simulink model "NNN_pick_and_place_without_camera"  (R2022b)
settings: Solver=ode4  StartTime=0.0  StopTime=inf  FixedStep=1/500  RelTol=1e-3  EnableMultiTasking=on
InitFcn:
  | % Positions
  | home = [0; 0.49; 0.45];
  | pick = [0.49; 0; 0.45];
  | place = [-0.3; -0.3; 0.05];
  | 
  | % Liste des cibles : On alterne juste entre Pick et Place
  | % Le format doit être : [x1 y1 z1; x2 y2 z2; ...]
  | waypoints = [pick'; place'];
  | 
  | % Vitesse désirée (m/s) - Remplace la durée fixe
  | robot_speed = 0.4;
  | 
  | % Temps de pause (secondes)
  | wait_time_home = 2; % Temps de repos avant le pick and place
  | wait_time_pick = 2 ;  % Temps pour attraper
  | wait_time_place = 1 ; % Temps pour déposer
  | 
  | wait_times = [wait_time_home, wait_time_pick, wait_time_place];
undefined symbols (not defined in the file): HIL, qc_get_step_size, waypoints
libraries: quarc_library x8
settings Model: SimulationMode=external  ExtModeTrigDuration=10000  Creator=fvranes  LastModifiedBy=QARM2
settings SolverCC: AlgebraicLoopSolver=TrustRegion  PositivePriorityOrder=on
settings DataIOCC: SaveOutput=off  SignalLogging=off  DSMLogging=off  SaveTime=off  ReturnWorkspaceOutputs=off
settings DebuggingCC: UnconnectedInputMsg=warning  UnconnectedOutputMsg=warning  UnconnectedLineMsg=warning  SFMachineParentedDataDiag=warning  ArithmeticOperatorsInVariantConditions=warning
settings ModelReferenceCC: EnableRefExpFcnMdlSchedulingChecks=on
settings SFSimCC: SimUseLocalCustomCode=off  CustomCodeUndefinedFunction=UseInterfaceOnly
settings RTWCC: Description=QUARC Win64 Target Using Toolchain  SystemTargetFile=quarc_win64.tlc  TemplateMakefile=quarc_default_tmf  RTWUseLocalCustomCode=off  Toolchain=QUARC win64 | nmake (64-bit Windows)  BuildConfiguration=Faster Runs
settings CodeAppCC: StateflowObjectComments=on
settings STFCustomTargetCC: TargetLangStandard=C99 (ISO)  ConcurrentExecutionCompliant=on  GRTInterface=on  UseToolchainInfoCompliant=on  SystemTargetFile=quarc_win64.tlc
settings GRTTargetCC: ParMdlRefBuildCompliant=off  CompOptLevelCompliant=off  CombineOutputUpdateFcns=off  MatFileLogging=off  CPPClassGenCompliant=off  GRTInterface=on  ExtMode=on  ExtModeMexFile=quarc_comm
settings ConfigComp: CovMetricSettings=dswe

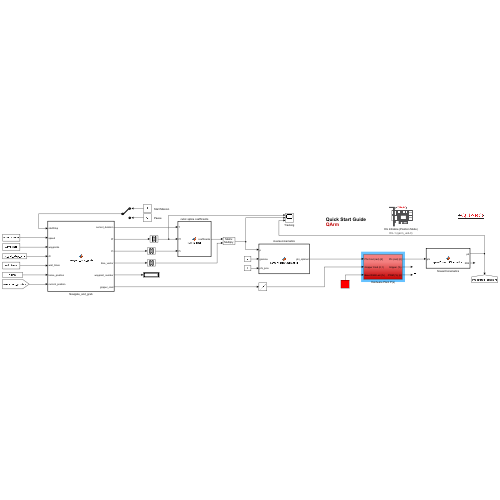
[thumbnail: Simulink's stored preview of the top-level diagram]
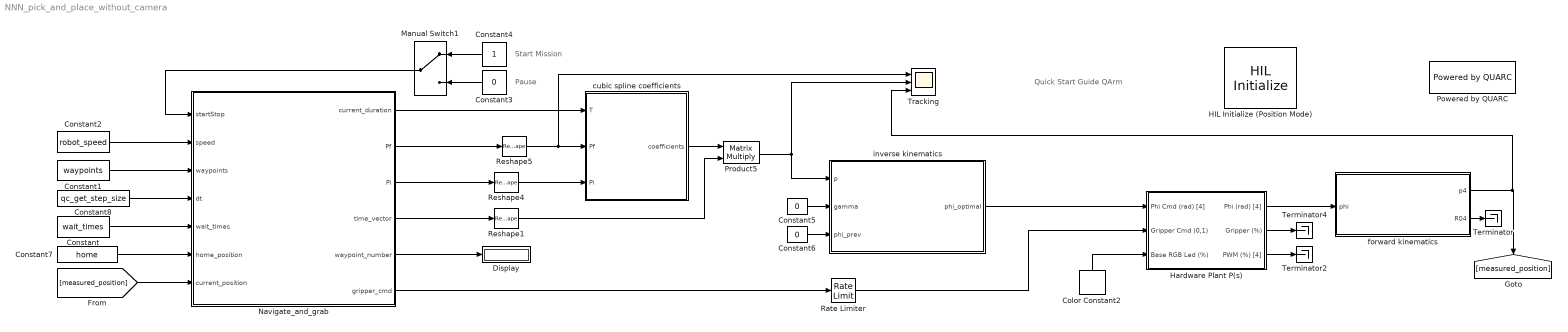
== system NNN_pick_and_place_without_camera ==
  note: Quick Start Guide
      | QArm
  note: Pause
  note: Start Mission
  Color Constant2 : quarc_library/Sources/Signals/Color Constant  color=[1 0 0]
      settings: SourceProductName=QUARC Targets
  Constant : Constant  Value=wait_times
  Constant1 : Constant  Value=waypoints  VectorParams1D=off
  Constant2 : Constant  Value=robot_speed
  Constant3 : Constant  Value=0
  Constant4 : Constant
  Constant5 : Constant  Value=0
  Constant6 : Constant  Value=0
  Constant7 : Constant  Value=home
  Constant8 : Constant  Value=qc_get_step_size
  Display : Display
  HIL Initialize (Position Mode) : quarc_library/Data Acquisition/Generic/Configuration/HIL Initialize  object_name=HIL-1  board_type=qarm_usb  board_number=0  board_options=j0_mode=0;j1_mode=0;j2_mode=0;j3_mode=0;gripper_mode=0;j0_profile_config=0;j0_profile_velocity=1.5708;j0_profile_acceleration=1.0472;j1_profile_config=0;j1_profile_velocity=1.5708;j1_profile_acceleration=1.0472;j2_profile_config=0;j2_profile_velocity=1.5708;j2_profile_acceleration=1.0472;j3_profile_config=0;j3_profile_velocity=1.5708;j3_profile_acceleration=1.0472;  exclusive=off  active=on  hardware_clocks=[0]  clock_modes=[]  initial_clock_frequencies=[]  set_clock_params_at_start=off  set_clock_params_at_switch_in=off  set_clock_frequencies_at_start=off  set_clock_frequencies_at_switch_in=off  analog_input_channels=[0:9]  analog_input_configurations=[]  analog_input_maximums=5  analog_input_minimums=0  set_analog_input_params_at_start=off  set_analog_input_params_at_switch_in=off  analog_output_channels=[]  analog_output_maximums=[]  analog_output_minimums=[]  initial_analog_outputs=[]  final_analog_outputs=[]  watchdog_analog_outputs=[]  set_analog_output_params_at_start=off  set_analog_output_params_at_switch_in=off  set_analog_outputs_at_start=off  set_analog_outputs_at_switch_in=off  set_analog_outputs_at_terminate=off  set_analog_outputs_at_switch_out=off  set_analog_outputs_on_watchdog=off  digital_input_channels=[]  digital_output_channels=[]  digital_output_configuration=[]  initial_digital_outputs=[0]  final_digital_outputs=[0]  watchdog_digital_outputs=[0]  set_digital_output_params_at_start=off  set_digital_output_params_at_switch_in=off  set_digital_outputs_at_start=on  set_digital_outputs_at_switch_in=off  set_digital_outputs_at_terminate=on  set_digital_outputs_at_switch_out=off  set_digital_outputs_on_watchdog=on  encoder_channels=[]  quadrature=[4]  encoder_filter_frequency=[]  initial_encoder_counts=[0]  set_encoder_params_at_start=off  set_encoder_params_at_switch_in=off  set_encoder_counts_at_start=on  set_encoder_counts_at_switch_in=off  pwm_channels=[]  pwm_modes=[0]  pwm_frequency=50  pwm_configuration=[0]  pwm_alignment=[0]  pwm_polarity=[1]  pwm_leading_deadband=[]  pwm_trailing_deadband=[]  initial_pwm_outputs=[0]  final_pwm_outputs=[0]  watchdog_pwm_outputs=[0]  set_pwm_params_at_start=on  set_pwm_params_at_switch_in=off  set_pwm_outputs_at_start=on  set_pwm_outputs_at_switch_in=off  set_pwm_outputs_at_terminate=on  set_pwm_outputs_at_switch_out=off  set_pwm_outputs_on_watchdog=on  other_output_channels=[1000:1004 11000:11008]  initial_other_outputs=[0]  final_other_outputs=[0]  watchdog_other_outputs=[0]  set_other_outputs_at_start=on  set_other_outputs_at_switch_in=off  set_other_outputs_at_terminate=on  set_other_outputs_at_switch_out=off  set_other_outputs_on_watchdog=on
  Hardware Plant P(s) : Subsystem
  Manual Switch1 : ManualSwitch
  Navigate_and_grab : MATLAB Function  TreatAsAtomicUnit=on
  Powered by QUARC : quarc_library/Logos/Powered by QUARC
  Product5 : Product  Multiplication=Matrix(*)
  Rate Limiter : RateLimiter  RisingSlewLimit=0.05
  Reshape1 : Reshape  OutputDimensionality=Column vector (2-D)
  Reshape4 : Reshape  OutputDimensionality=Column vector (2-D)
  Reshape5 : Reshape  OutputDimensionality=Column vector (2-D)
  Terminator : Terminator
  Terminator2 : Terminator
  Terminator4 : Terminator
  Tracking : Scope  NumInputPorts=3
  cubic spline coefficients : MATLAB Function  TreatAsAtomicUnit=on
  forward kinematics : MATLAB Function  TreatAsAtomicUnit=on
  inverse kinematics : MATLAB Function  TreatAsAtomicUnit=on
  wires:
  forward kinematics/2(R04) -> Terminator/1
  Hardware Plant P(s)/1(Phi (rad) [4]) -> forward kinematics/1(phi)
  Color Constant2/1 -> Hardware Plant P(s)/3(Base RGB Led (%))
  Rate Limiter/1 -> Hardware Plant P(s)/2(Gripper Cmd (0,1))
  Hardware Plant P(s)/3(PWM (%) [4]) -> Terminator2/1
  Hardware Plant P(s)/2(Gripper (%)) -> Terminator4/1
  inverse kinematics/1(phi_optimal) -> Hardware Plant P(s)/1(Phi Cmd (rad) [4])
  Constant1/1 -> Navigate_and_grab/3(waypoints)
  Navigate_and_grab/3(Pi) -> Reshape4/1
  Constant4/1 -> Manual Switch1/1
  Navigate_and_grab/4(time_vector) -> Reshape1/1
  cubic spline coefficients/1(coefficients) -> Product5/1
  Constant8/1 -> Navigate_and_grab/4(dt)
  Manual Switch1/1 -> Navigate_and_grab/1(startStop)
  Navigate_and_grab/2(Pf) -> Reshape5/1
  Constant3/1 -> Manual Switch1/2
  Constant2/1 -> Navigate_and_grab/2(speed)
  Reshape1/1 -> Product5/2
  Reshape4/1 -> cubic spline coefficients/3(Pi)
  Navigate_and_grab/5(waypoint_number) -> Display/1
  Reshape5/1 -> Tracking/1, cubic spline coefficients/2(Pf)
  Product5/1 -> Tracking/2, inverse kinematics/1(p)
  forward kinematics/1(p4) -> [measured_position], Tracking/3
  Constant5/1 -> inverse kinematics/2(gamma)
  Navigate_and_grab/1(current_duration) -> cubic spline coefficients/1(T)
  Navigate_and_grab/6(gripper_cmd) -> Rate Limiter/1
  Constant/1 -> Navigate_and_grab/5(wait_times)
  Constant7/1 -> Navigate_and_grab/6(home_position)
  [measured_position] -> Navigate_and_grab/7(current_position)
  Constant6/1 -> inverse kinematics/3(phi_prev)

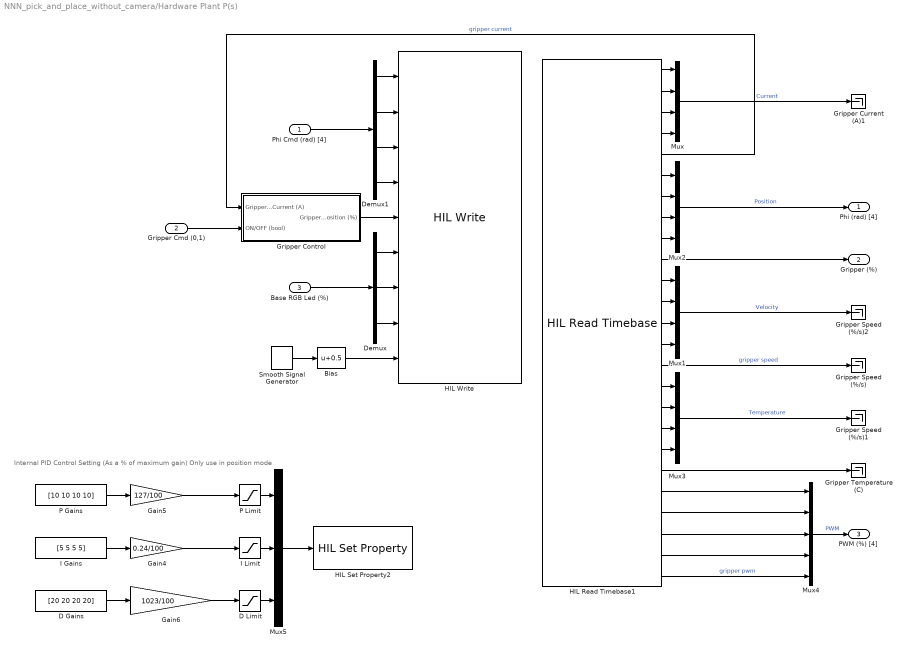
== system NNN_pick_and_place_without_camera/Hardware Plant P(s) ==
  note: Internal PID Control Setting (As a % of maximum gain)
      | Only use in position mode
  Phi Cmd (rad) [4] : Inport
  Gripper Cmd (0,1) : Inport  Port=2
  Base RGB Led (%) : Inport  Port=3
  Bias : Bias  Bias=0.5  SaturateOnIntegerOverflow=off
  D Gains : Constant  Value=[20 20 20 20]
  D Limit : Saturate  UpperLimit=[1023 1023 1023 1023]  LowerLimit=[0 0 0 0]
  Demux : Demux  Outputs=3
  Demux1 : Demux
  Gain4 : Gain  Gain=0.24/100
  Gain5 : Gain  Gain=127/100
  Gain6 : Gain  Gain=1023/100
  Gripper Control : Subsystem
  Gripper Current (A)1 : Terminator
  Gripper Speed (%/s) : Terminator
  Gripper Speed (%/s)1 : Terminator
  Gripper Speed (%/s)2 : Terminator
  Gripper Temperature (C) : Terminator
  HIL Read Timebase1 : quarc_library/Data Acquisition/Generic/Timebases/HIL Read Timebase  object_name=HIL-1  clock=0  analog_channels=[5:9]  encoder_channels=[]  digital_channels=[]  other_channels=[1000:1004 3000:3004 10000:10004 11000:11004]  active=on  vector_output=off  data_type_mode=Inherit via back propagation  encoder_data_type=double  digital_data_type=boolean  overflow_mode=Error on overflow  samples_in_buffer=max(ceil(1/qc_get_step_size), 1)
  HIL Set Property2 : quarc_library/Data Acquisition/Generic/Configuration/HIL Set Property  object_name=HIL-1  property_type=2  property_codes=[128:131 133:136 138:141]  property_source=2  property_value_num=0  set_at_start=on  sample_time=-1  active=off
      settings: AttributesFormatString=(%<object_name>)  SourceProductName=QUARC Targets
  HIL Write : quarc_library/Data Acquisition/Generic/Immediate I//O/HIL Write  object_name=HIL-1  analog_channels=[]  pwm_channels=[]  digital_channels=[]  other_channels=[1000:1004 11005:11008]  sample_time=-1  active=on  vector_input=off
  I Gains : Constant  Value=[5 5 5 5]
  I Limit : Saturate  UpperLimit=[0.24 0.24 0.24 0.24]  LowerLimit=[0 0 0 0]
  Mux{,1..3} (4 alike) : Mux
  Mux4 : Mux  Inputs=5
  Mux5 : Mux  Inputs=3
  P Gains : Constant  Value=[10 10 10 10]
  P Limit : Saturate  UpperLimit=[127 127 127 127]  LowerLimit=[0 0 0 0]
  Smooth Signal Generator : quarc_library/Sources/Signals/Smooth Signal Generator  signal_type=Sine  source=Internal (dialog parameters)  amplitude=0.5  frequency=60/72  initial_phase=0  sample_time=qc_get_step_size  output_cos=off
      settings: SourceProductName=QUARC Targets
  Phi (rad) [4] : Outport  VectorParamsAs1DForOutWhenUnconnected=off
  Gripper (%) : Outport  Port=2  VectorParamsAs1DForOutWhenUnconnected=off
  PWM (%) [4] : Outport  Port=3  VectorParamsAs1DForOutWhenUnconnected=off
  wires:
  HIL Read Timebase1/10 -> Gripper (%)/1
  Mux4/1 -> PWM (%) [4]/1  "PWM"
  HIL Read Timebase1/25 -> Mux4/5  "gripper pwm"
  HIL Read Timebase1/24 -> Mux4/4
  HIL Read Timebase1/23 -> Mux4/3
  HIL Read Timebase1/22 -> Mux4/2
  HIL Read Timebase1/21 -> Mux4/1
  Mux2/1 -> Phi (rad) [4]/1  "Position"
  Phi Cmd (rad) [4]/1 -> Demux1/1
  Demux1/4 -> HIL Write/4
  Demux1/3 -> HIL Write/3
  Demux1/2 -> HIL Write/2
  Demux1/1 -> HIL Write/1
  Base RGB Led (%)/1 -> Demux/1
  Mux3/1 -> Gripper Speed (%/s)1/1  "Temperature"
  Mux1/1 -> Gripper Speed (%/s)2/1  "Velocity"
  Mux/1 -> Gripper Current (A)1/1  "Current"
  HIL Read Timebase1/20 -> Gripper Temperature (C)/1
  HIL Read Timebase1/1 -> Mux/1
  HIL Read Timebase1/2 -> Mux/2
  HIL Read Timebase1/13 -> Mux1/3
  Demux/2 -> HIL Write/7
  HIL Read Timebase1/19 -> Mux3/4
  Demux/1 -> HIL Write/6
  HIL Read Timebase1/11 -> Mux1/1
  HIL Read Timebase1/16 -> Mux3/1
  HIL Read Timebase1/17 -> Mux3/2
  HIL Read Timebase1/3 -> Mux/3
  Demux/3 -> HIL Write/8
  HIL Read Timebase1/15 -> Gripper Speed (%/s)/1  "gripper speed"
  HIL Read Timebase1/5 -> Gripper Control/1(Gripper Current (A))  "gripper current"
  HIL Read Timebase1/7 -> Mux2/2
  HIL Read Timebase1/4 -> Mux/4
  HIL Read Timebase1/12 -> Mux1/2
  HIL Read Timebase1/8 -> Mux2/3
  HIL Read Timebase1/18 -> Mux3/3
  HIL Read Timebase1/6 -> Mux2/1
  HIL Read Timebase1/9 -> Mux2/4
  HIL Read Timebase1/14 -> Mux1/4
  Gripper Control/1(Gripper Position (%)) -> HIL Write/5
  Gripper Cmd (0,1)/1 -> Gripper Control/2(ON/OFF (bool))
  Smooth Signal Generator/1 -> Bias/1
  Bias/1 -> HIL Write/9
  P Limit/1 -> Mux5/1
  D Gains/1 -> Gain6/1
  D Limit/1 -> Mux5/3
  P Gains/1 -> Gain5/1
  Mux5/1 -> HIL Set Property2/1
  I Limit/1 -> Mux5/2
  Gain6/1 -> D Limit/1
  Gain5/1 -> P Limit/1
  Gain4/1 -> I Limit/1
  I Gains/1 -> Gain4/1

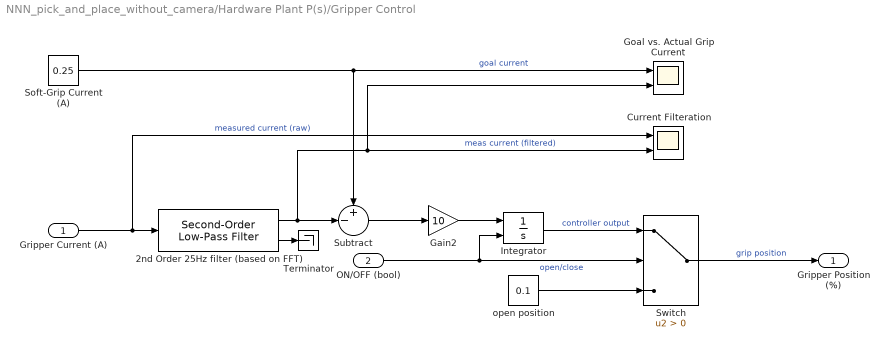
== system NNN_pick_and_place_without_camera/Hardware Plant P(s)/Gripper Control ==
  Gripper Current (A) : Inport
  ON/OFF (bool) : Inport  Port=2
  2nd Order 25Hz filter (based on FFT) : quarc_library/Continuous/Second-Order Low-Pass Filter  params_source=Internal (dialog parameters)  input_width=25*2*pi  input_zeta=1  input_init=0
  Current Filteration : Scope  NumInputPorts=2
  Gain2 : Gain  Gain=10
  Goal vs. Actual Grip Current : Scope  NumInputPorts=2
  Integrator : Integrator  ExternalReset=either  InitialCondition=0.1  LimitOutput=on  UpperSaturationLimit=0.9  LowerSaturationLimit=0.1
  Soft-Grip Current (A) : Constant  Value=0.25
  Subtract : Sum  Inputs=+-|
  Switch : Switch  Criteria=u2 > Threshold  SaturateOnIntegerOverflow=off  InputSameDT=off
  Terminator : Terminator
  open position : Constant  Value=0.1
  Gripper Position (%) : Outport  VectorParamsAs1DForOutWhenUnconnected=off
  wires:
  Gripper Current (A)/1 -> 2nd Order 25Hz filter (based on FFT)/1, Current Filteration/1  "measured current (raw)"
  ON/OFF (bool)/1 -> Switch/2, Integrator/2  "open/close"
  open position/1 -> Switch/3
  Switch/1 -> Gripper Position (%)/1  "grip position"
  Soft-Grip Current (A)/1 -> Subtract/1, Goal vs. Actual Grip Current/1  "goal current"
  2nd Order 25Hz filter (based on FFT)/1 -> Subtract/2, Current Filteration/2, Goal vs. Actual Grip Current/2  "meas current (filtered)"
  Subtract/1 -> Gain2/1
  Integrator/1 -> Switch/1  "controller output"
  Gain2/1 -> Integrator/1
  2nd Order 25Hz filter (based on FFT)/2 -> Terminator/1

== matlab function NNN_pick_and_place_without_camera/Navigate_and_grab ==
  data: startStop input; current_duration output; speed input; waypoints input; Pf output; dt input; wait_times input; home_position input; current_position input; Pi output; time_vector output; waypoint_number output; gripper_cmd output
function [current_duration, Pf, Pi, time_vector, waypoint_number, gripper_cmd] = navigate_and_grab(startStop, speed, waypoints, dt, wait_times, home_position, current_position)
    % MODIFICATION : Une seule entrée 'wait_times' à la fin au lieu de 3 séparées.
    % On suppose que wait_times = [Temps_Home, Temps_Pick, Temps_Place]

    %% Rising slew rate est la vitesse de fermeture
    %%falling slew rate est la vitesse d'ouverture

    %% 0. Lecture des temps (pour lisibilité)
    % C'est plus propre de les nommer ici que d'utiliser wait_times(1) partout
    TIME_HOME  = wait_times(1);
    TIME_PICK  = wait_times(2);
    TIME_PLACE = wait_times(3);

    %% 1. Initialisation
    persistent state          % 0:Vers Home, 1:Vers Waypoint, 2:Pause
    persistent p_start p_end  % Points
    persistent target_idx     % Index cible
    persistent t_clock        % Chrono
    persistent t_travel       % Durée voyage
    persistent t_wait         % Durée pause
    persistent grip_state     % État pince
    
    POSITION_TOLERANCE = 0.04; % 5 cm

    if isempty(state)
        state = 0;          
        p_start = current_position; 
        p_end = home_position;      
        target_idx = 1;     
        t_clock = 0;
        
        dist = norm(p_end - p_start);
        if speed > 0
            t_travel = dist / speed;
        else
            t_travel = 5; 
        end
        t_travel = max(t_travel, 0.05);
        
        t_wait = 0;
        grip_state = 0;     
    end

    %% 2. Machine à États
    if startStop
        switch state
            
            case 0 % --- INIT : VERS HOME ---
                t_clock = t_clock + dt;
                current_error = norm(current_position - p_end);
                
                if t_clock >= t_travel && current_error < POSITION_TOLERANCE
                    % Arrivé Home -> PAUSE
                    state = 2; 
                    t_clock = 0;
                    p_start = p_end; 
                    
                    t_wait = TIME_HOME; % On utilise la valeur extraite du vecteur
                    
                    target_idx = 0; 
                    grip_state = 0; 
                end
                
            case 1 % --- MOUVEMENT (Cycle) ---
                t_clock = t_clock + dt;
                current_error = norm(current_position - p_end);

                if t_clock >= t_travel && current_error < POSITION_TOLERANCE
                    state = 2; 
                    t_clock = 0;
                    p_start = p_end; 
                    
                    if target_idx == 1 
                        % Pick
                        t_wait = TIME_PICK; % Valeur du vecteur
                        grip_state = 1; 
                    else 
                        % Place
                        t_wait = TIME_PLACE; % Valeur du vecteur
                        grip_state = 0; 
                    end
                end

            case 2 % --- PAUSE ---
                t_clock = t_clock + dt;
                
                if t_clock >= t_wait
                    % Fin de pause -> On repart
                    state = 1; 
                    t_clock = 0;
                    p_start = p_end; 
                    
                    target_idx = target_idx + 1;
                    [num_pts, ~] = size(waypoints);
                    if target_idx > num_pts
                        target_idx = 1; 
                    end
                    p_end = waypoints(target_idx, :)';
                    
                    dist = norm(p_end - p_start);
                    t_travel = max(dist / speed, 0.05);
                end
        end
    end

    %% 3. Sorties
    waypoint_number = target_idx;
    current_duration = t_travel; 
    gripper_cmd = grip_state;

    if state == 2 
        Pi = p_end;
        Pf = p_end;
        time_vector = [1; 0; 0; 0]; 
    else
        Pi = p_start;
        Pf = p_end;
        t_spline = min(t_clock, t_travel);
        time_vector = [1; t_spline; t_spline^2; t_spline^3];
    end
end

== matlab function NNN_pick_and_place_without_camera/cubic spline coefficients ==
  data: T input; coefficients output; Pf input; Pi input
function coefficients = cubicSpline(T, Pf, Pi)
    
    % --- REGLAGE AGRESSIVITE ---
    % 0.0 = Démarrage ultra doux (Ton code actuel, Vitesse Initiale = 0)
    % 0.1 = Démarrage un peu plus vif
    % 0.3 = Démarrage rapide (Attention au petit "choc" mécanique)
    % 1.0 = Démarrage brutal (Vitesse constante tout le long, a-coup violent)
    aggressiveness = 0.2; 
    
    % Calcul de la vitesse moyenne nécessaire pour faire le trajet
    % V_moyenne = Distance / Temps
    if T > 0.001
        V_avg = (Pf - Pi) / T;
    else
        V_avg = [0;0;0];
    end
    
    % On définit la Vitesse Initiale (Vi) et Finale (Vf)
    % Au lieu de 0, on met une fraction de la vitesse moyenne
    Vi = V_avg * aggressiveness;
    Vf = [0;0;0]; % On veut quand même s'arrêter doucement à la fin !

    % --- CALCUL DES COEFFICIENTS (Formule Générale) ---
    % a0 = Position Initiale
    a0 = Pi;
    
    % a1 = Vitesse Initiale
    a1 = Vi;
    
    % a2 = Accélération (Formule adaptée pour Vi non nulle)
    % Formule mathématique : (3*DeltaP - 2*Vi*T - Vf*T) / T^2
    a2 = (3*(Pf - Pi) - 2*Vi*T - Vf*T) / (T^2);
    
    % a3 = Jerk (Formule adaptée pour Vi non nulle)
    % Formule mathématique : (-2*DeltaP + (Vi + Vf)*T) / T^3
    a3 = (-2*(Pf - Pi) + (Vi + Vf)*T) / (T^3);

    % Output as coloumns
    coefficients = [a0, a1, a2, a3];
end

== matlab function NNN_pick_and_place_without_camera/forward kinematics ==
  data: phi input; p4 output; R04 output
function [p4, R04] = qarmForwardKinematics(phi)

%% QUANSER_ARM_FPK
% v 4.0 - 4th June 2020

% REFERENCE: 
% Chapter 3. Forward Kinematics
% Robot Dynamics and Control 
% Spong, Vidyasagar
% 1989

% INPUTS:
% phi     : Alternate joint angles vector 4 x 1

% OUTPUTS:
% p4      : End-effector frame {4} position vector expressed in base frame {0}
% R04     : rotation matrix from end-effector frame {4} to base frame {0}

%% Manipulator parameters:
L1 = 0.1400;
L2 = 0.3500;
L3 = 0.0500;
L4 = 0.2500;
L5 = 0.1500;

%% Alternate parameters
l1 = L1;
l2 = sqrt(L2^2 + L3^2);
l3 = L4 + L5;
beta = atan(L3/L2);

%% From phi space to theta space 
theta = phi;
theta(1) = phi(1);
theta(2) = phi(2) + beta - pi/2;
theta(3) = phi(3) - beta;
theta(4) = phi(4);

%% Transformation matrices for all frames:

% T{i-1}{i} = quanser_arm_DH(  a, alpha,  d,     theta );
        T01 = quanser_arm_DH(  0, -pi/2, l1,  theta(1) );
        T12 = quanser_arm_DH( l2,     0,  0,  theta(2) );
        T23 = quanser_arm_DH(  0, -pi/2,  0,  theta(3) );
        T34 = quanser_arm_DH(  0,     0, l3,  theta(4) );

        T02 = T01*T12;
        T03 = T02*T23;
        T04 = T03*T34;

%% Position of end-effector Transformation

% Extract the Position vector 
% p1   = T01(1:3,4);
% p2   = T02(1:3,4);
% p3   = T03(1:3,4);
p4   = T04(1:3,4);

% Extract the Rotation matrix
% R01 = T01(1:3,1:3);
% R02 = T02(1:3,1:3);
% R03 = T03(1:3,1:3);
R04 = T04(1:3,1:3);

end

function T = quanser_arm_DH(a,alpha,d,theta)

%% QUANSER_ARM_DH
% v 1.0 - 26th March 2019

% REFERENCE: 
% Chapter 3. Forward and Inverse Kinematics
% Robot Modeling and Control 
% Spong, Hutchinson, Vidyasagar
% 2006

% INPUTS:
% a       :   translation  : along : x_{i}   : from : z_{i-1} : to : z_{i}
% alpha   :      rotation  : about : x_{i}   : from : z_{i-1} : to : z_{i}
% d       :   translation  : along : z_{i-1} : from : x_{i-1} : to : x_{i}
% theta   :      rotation  : about : z_{i-1} : from : x_{i-1} : to : x_{i}
% NOTE: Standard DH Parameters

% OUTPUTS:
% T       : transformation                   : from :     {i} : to : {i-1}

%%
% Rotation Transformation about z axis by theta
T_R_z = [cos(theta) -sin(theta) 0 0;
         sin(theta)  cos(theta) 0 0;
                  0           0 1 0;
                  0           0 0 1];
     
% Translation Transformation along z axis by d
T_T_z = [1 0 0 0;
         0 1 0 0;
         0 0 1 d;
         0 0 0 1];

% Translation Transformation along x axis by a
T_T_x = [1 0 0 a;
         0 1 0 0;
         0 0 1 0;
         0 0 0 1];

% Rotation Transformation about x axis by alpha
T_R_x = [1          0           0 0;
         0 cos(alpha) -sin(alpha) 0;
         0 sin(alpha)  cos(alpha) 0;
         0          0           0 1];

% For a transformation FROM frame {i} TO frame {i-1}: A
T = T_R_z*T_T_z*T_T_x*T_R_x;

end

== matlab function NNN_pick_and_place_without_camera/inverse kinematics ==
  data: p input; gamma input; phi_optimal output; phi_prev input
function phi_optimal = qarmInverseKinematics(p, gamma, phi_prev)

%% QUANSER_ARM_IPK
% v 4.0 - 4th June 2020

% REFERENCE: 
% Chapter 4. Inverse Kinematics
% Robot Dynamics and Control 
% Spong, Vidyasagar
% 1989

% INPUTS:
% p        : end-effector position vector expressed in base frame {0}
% gamma    : wrist rotation angle gamma

% OUTPUTS:
% phi_optimal : Best solution depending on phi_prev
% phi         : All four Inverse Kinematics solutions as a 4x4 matrix. 
%               Each col is a solution.

%% Manipulator parameters:
L1 = 0.1400;
L2 = 0.3500;
L3 = 0.0500;
L4 = 0.2500;
L5 = 0.1500;
beta = atan(L3/L2);

%% Alternate parameters
lambda1 = L1;
lambda2 = sqrt(L2^2 + L3^2);
lambda3 = L4 + L5;

%% Initialization
theta   = zeros(4, 4);
phi = zeros(4, 4);

%% Joint angle 2 and 3: 
% Equations:
    % lambda2 cos(theta2) + (-lambda3) sin(theta2 + theta3) = sqrt(x^2 + y^2)
    %   A     cos( 2    ) +     C      sin(   2   +    3  ) =    D
    
    % lambda2 sin(theta2) - (-lambda3) cos(theta2 + theta3) = lambda1 - z
    %   A     sin( 2    ) -     C      cos(   2   +    3  ) =    H

% Solution:
    A = lambda2;
    C = -lambda3;
    H =  lambda1 - p(3);
    D1 = -sqrt(p(1)^2 + p(2)^2);
    D2 = sqrt(p(1)^2 + p(2)^2);
    F = (D1^2 + H^2 - A^2 - C^2)/(2*A);

    theta(3,1) = 2*atan2( C + sqrt(C^2 - F^2) , F );
	theta(3,2) = 2*atan2( C - sqrt(C^2 - F^2) , F );
    theta(3,3) = 2*atan2( C + sqrt(C^2 - F^2) , F );
	theta(3,4) = 2*atan2( C - sqrt(C^2 - F^2) , F );

    M = A + C*sin(theta(3,1));
    N = -C*cos(theta(3,1));
    cos_term = (D1*M + H*N)/(M^2 + N^2);
    sin_term = (H - N*cos_term)/(M);
    theta(2,1) = atan2(sin_term, cos_term);

    M = A + C*sin(theta(3,2));
    N = -C*cos(theta(3,2));
    cos_term = (D1*M + H*N)/(M^2 + N^2);
    sin_term = (H - N*cos_term)/(M);
    theta(2,2) = atan2(sin_term, cos_term);

    M = A + C*sin(theta(3,3));
    N = -C*cos(theta(3,3));
    cos_term = (D2*M + H*N)/(M^2 + N^2);
    sin_term = (H - N*cos_term)/(M);
    theta(2,3) = atan2(sin_term, cos_term);

    M = A + C*sin(theta(3,4));
    N = -C*cos(theta(3,4));
    cos_term = (D2*M + H*N)/(M^2 + N^2);
    sin_term = (H - N*cos_term)/(M);
    theta(2,4) = atan2(sin_term, cos_term);


%% Joint angle 1:
% Equation:
    % y / x = tan(theta1);

% Solution
    theta(1,1) = atan2( p(2)/( lambda2 * cos( theta(2,1) ) - lambda3 * sin( theta(2,1) + theta(3,1) ) ) , p(1)/(  lambda2 * cos( theta(2,1) ) - lambda3 * sin( theta(2,1) + theta(3,1) )  ) );
    theta(1,2) = atan2( p(2)/( lambda2 * cos( theta(2,2) ) - lambda3 * sin( theta(2,2) + theta(3,2) ) ) , p(1)/(  lambda2 * cos( theta(2,2) ) - lambda3 * sin( theta(2,2) + theta(3,2) )  ) );
    theta(1,3) = atan2( p(2)/( lambda2 * cos( theta(2,3) ) - lambda3 * sin( theta(2,3) + theta(3,3) ) ) , p(1)/(  lambda2 * cos( theta(2,3) ) - lambda3 * sin( theta(2,3) + theta(3,3) )  ) );
    theta(1,4) = atan2( p(2)/( lambda2 * cos( theta(2,4) ) - lambda3 * sin( theta(2,4) + theta(3,4) ) ) , p(1)/(  lambda2 * cos( theta(2,4) ) - lambda3 * sin( theta(2,4) + theta(3,4) )  ) );
    
%% Remap theta back to phi
% phi(1) = theta(1);
% phi(2) = theta(2) - beta + pi/2;
% phi(3) = theta(3) + beta;
% phi(4) = theta(4);

phi(1,:) = theta(1,:);
phi(2,:) = theta(2,:) - beta + pi/2;
phi(3,:) = theta(3,:) + beta;
phi(4,:) = gamma;

phi = mod(phi + pi, 2*pi) - pi;

phi_optimal = phi(:,1);
if (norm(phi_optimal - phi_prev) > norm(phi(:,2) - phi_prev)) || (check_joint_limits(phi_optimal))
    phi_optimal = phi(:,2);
end
if (norm(phi_optimal - phi_prev) > norm(phi(:,3) - phi_prev)) || (check_joint_limits(phi_optimal))
    phi_optimal = phi(:,3);
end
if (norm(phi_optimal - phi_prev) > norm(phi(:,4) - phi_prev)) || (check_joint_limits(phi_optimal))
    phi_optimal = phi(:,4);
end
if (check_joint_limits(phi_optimal))
    phi_optimal = [0;0;0;0];
end

end

function flag = check_joint_limits(phi)
    flag = 0;
    if phi(1) > 170*pi/180 || phi(1) < -170*pi/180 ...
        || phi(2) > 80*pi/180 || phi(2) < -80*pi/180 ...
        || phi(3) > 75*pi/180 || phi(3) < -95*pi/180 ...
        || phi(4) > 160*pi/180 || phi(4) < -160*pi/180
    flag = 1;
    end
end
